simulink model "Neurofeedback_PID_WithoutFNIRS.slx"  (R2021b)
settings: Solver=ode23tb  StartTime=0.0  StopTime=30  FixedStep=0.09  RelTol=1e-8
libraries: slpidlib x1
settings Model: Creator=mdls3  LastModifiedBy=mariodelossantos
settings SolverCC: ZeroCrossControl=EnableAll
settings DebuggingCC: UnderSpecifiedDimensionMsg=warning

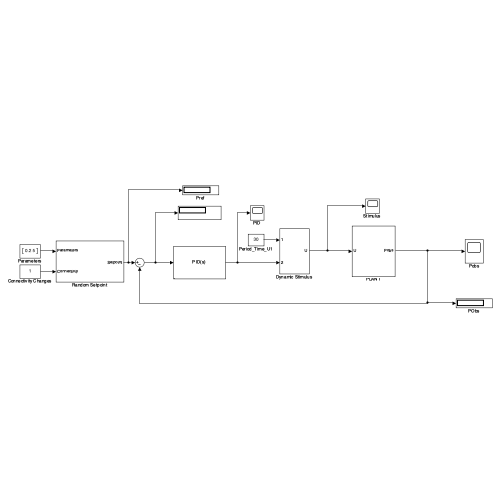
[thumbnail: Simulink's stored preview of the top-level diagram]
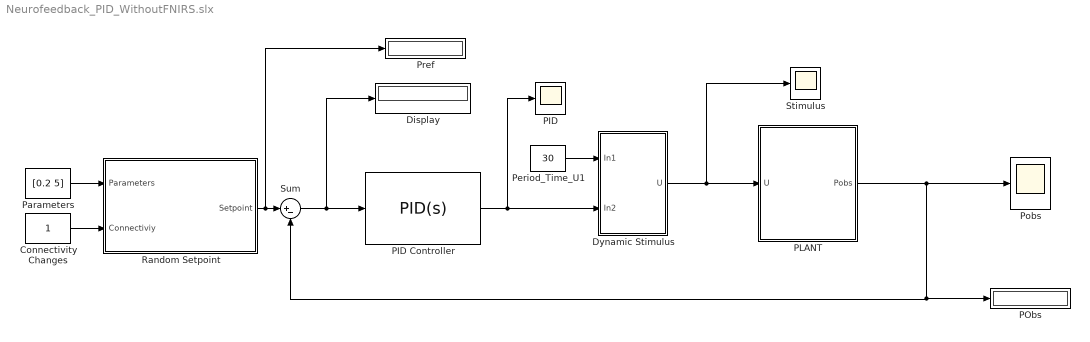
== system Neurofeedback_PID_WithoutFNIRS.slx ==
  Connectivity Changes : Constant
  Display : Display
  Dynamic Stimulus : Subsystem
  PID : Scope
  PID Controller : slpidlib/PID Controller  Controller=PID  Form=Ideal  TimeDomain=Continuous-time  UseExternalTs=off  SampleTime=-1  IntegratorMethod=Forward Euler  FilterMethod=Forward Euler  ControllerParametersSource=internal  P=0.87  I=0.1525  D=0.105  UseFilter=on  N=100  TunerSelectOption=Transfer Function Based (PID Tuner App)  InitialConditionSource=internal  InitialConditionForIntegrator=1  InitialConditionForFilter=0  DifferentiatorICPrevScaledInput=0  ExternalReset=none  TrackingMode=off  Kt=1  LimitOutput=off  SatLimitsSource=internal  UpperSaturationLimit=inf  LowerSaturationLimit=-inf  LinearizeAsGain=on  AntiWindupMode=none  Kb=1  POutMin=[]  POutMax=[]  IOutMin=[]  IOutMax=[]  DOutMin=[]  DOutMax=[]  NOutMin=[]  NOutMax=[]  SumOutMin=[]  SumOutMax=[]  SaturationOutMin=[]  SaturationOutMax=[]  PParamMin=[]  PParamMax=[]  IParamMin=[]  IParamMax=[]  DParamMin=[]  DParamMax=[]  NParamMin=[]  NParamMax=[]  KbParamMin=[]  KbParamMax=[]  KtParamMin=[]  KtParamMax=[]  KbOutMin=[]  KbOutMax=[]  KtOutMin=[]  KtOutMax=[]  IntegratorOutMin=[]  IntegratorOutMax=[]  FilterOutMin=[]  FilterOutMax=[]  SumI1OutMin=[]  SumI1OutMax=[]  SumI2OutMin=[]  SumI2OutMax=[]  SumI3OutMin=[]  SumI3OutMax=[]  SumI4OutMin=[]  SumI4OutMax=[]  SumDOutMin=[]  SumDOutMax=[]  DifferentiatorOutMin=[]  DifferentiatorOutMax=[]  FilterDiffOutCoefMin=[]  FilterDiffOutCoefMax=[]  ReciprocalOutMin=[]  ReciprocalOutMax=[]  SumDenOutMin=[]  SumDenOutMax=[]  SumNumOutMin=[]  SumNumOutMax=[]  DivideOutMin=[]  DivideOutMax=[]  UdiffTsProdOutMin=[]  UdiffTsProdOutMax=[]  NTsProdOutMin=[]  NTsProdOutMax=[]  UintegralTsProdOutMin=[]  UintegralTsProdOutMax=[]  UngainTsProdOutMin=[]  UngainTsProdOutMax=[]  IntegratorContinuousStateAttributes=''  IntegratorStateMustResolveToSignalObject=off  IntegratorRTWStateStorageClass=Auto  FilterContinuousStateAttributes=''  FilterStateMustResolveToSignalObject=off  FilterRTWStateStorageClass=Auto  ParallelPVariant=Passthrough  IdealPVariant=InternalParameters  IVariant=InternalParameters  DVariant=InternalParameters  IntegratorVariant=Continuous  SatVariant=Disabled  AWVariant=Passthrough  PCopyVariant=Disabled  TRVariant=Disabled  FdbkBlocksVariant=Forward  IdealPFdbkVariant=Disabled  SatFdbkVariant=Disabled  DerivativeFilterVariant=ContFilter  NVariant=InternalParameters  NCopyVariant=Disabled  FilterICVariant=InternalICsFilter  IntegratorICVariant=InternalICs  ExternalResetVariant=Disabled  TRSumVariant=Passthrough  SumFdbkVariant=Disabled  SumVariant=Sum_PID  TsampFilterVariant=InternalTs  TsampNgainVariant=Passthrough  TsampIntegralVariant=Passthrough  ExternalSaturationOutDataTypeStr=Inherit: Same as second input
  PLANT : Subsystem
  PObs : Display
  Parameters : Constant  Value=[0.2 5]
  Period_Time_U1 : Constant  Value=30
  Pobs : Scope
  Pref : Display
  Random Setpoint : Subsystem
  Stimulus : Scope
  Sum : Sum  Inputs=|+-
  wires:
  Period_Time_U1/1 -> Dynamic Stimulus/1(In1)
  Dynamic Stimulus/1(U) -> Stimulus/1, PLANT/1(U)
  PID Controller/1 -> Dynamic Stimulus/2(In2), PID/1
  Sum/1 -> PID Controller/1, Display/1
  PLANT/1(Pobs) -> Pobs/1, Sum/2, PObs/1
  Parameters/1 -> Random Setpoint/1(Parameters)
  Random Setpoint/1(Setpoint) -> Pref/1, Sum/1
  Connectivity Changes/1 -> Random Setpoint/2(Connectiviy)

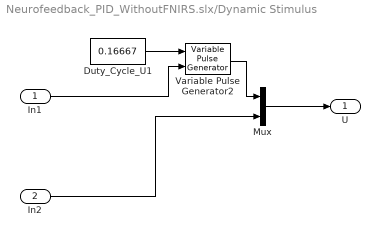
== system Neurofeedback_PID_WithoutFNIRS.slx/Dynamic Stimulus ==
  In1 : Inport
  In2 : Inport  Port=2
  Duty_Cycle_U1 : Constant  Value=0.16667  OutMin=[0]  OutMax=[0.8]
  Mux : Mux  Inputs=2
  Variable Pulse Generator2 : VariablePulseGenerator  RunAtFixedTimeIntervals=on  SampleTime=1/10.4
  U : Outport
  wires:
  In1/1 -> Variable Pulse Generator2/2
  Mux/1 -> U/1
  Variable Pulse Generator2/1 -> Mux/1
  Duty_Cycle_U1/1 -> Variable Pulse Generator2/1
  In2/1 -> Mux/2

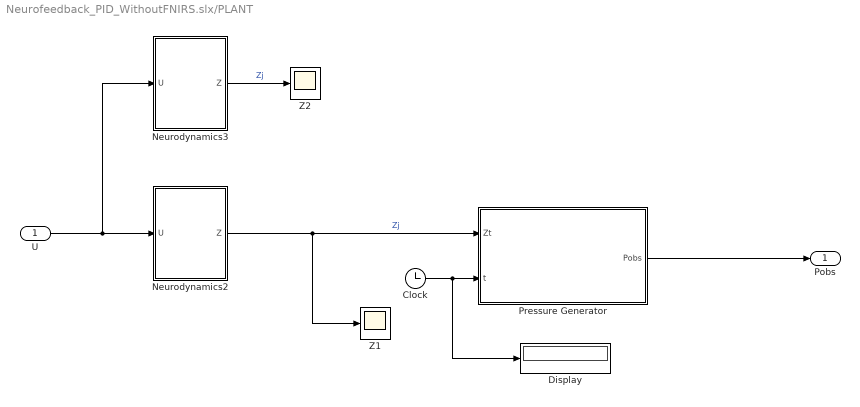
== system Neurofeedback_PID_WithoutFNIRS.slx/PLANT ==
  U : Inport
  Clock : Clock
  Display : Display
  Neurodynamics2 : Subsystem
  Neurodynamics3 : Subsystem
  Pressure Generator : MATLAB Function  TreatAsAtomicUnit=on
  Z1 : Scope
  Z2 : Scope
  Pobs : Outport
  wires:
  Clock/1 -> Display/1, Pressure Generator/2(t)
  Pressure Generator/1(Pobs) -> Pobs/1
  Neurodynamics2/1(Z) -> Z1/1, Pressure Generator/1(Zt)  "Zj"
  U/1 -> Neurodynamics3/1(U), Neurodynamics2/1(U)
  Neurodynamics3/1(Z) -> Z2/1  "Zj"

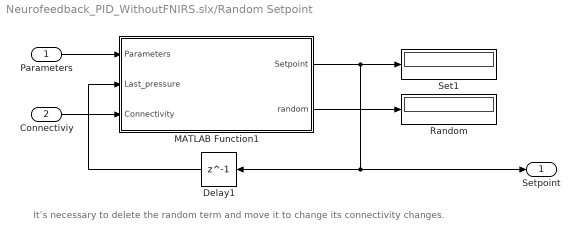
== system Neurofeedback_PID_WithoutFNIRS.slx/Random Setpoint ==
  note: It’s necessary to delete the random term and move it to change its connectivity changes.
  Parameters : Inport
  Connectiviy : Inport  Port=2
  Delay1 : Delay  DelayLength=1  InitialCondition=0
  MATLAB Function1 : MATLAB Function  TreatAsAtomicUnit=on
  Random : Display
  Set1 : Display
  Setpoint : Outport
  wires:
  Parameters/1 -> MATLAB Function1/1(Parameters)
  MATLAB Function1/2(random) -> Random/1
  MATLAB Function1/1(Setpoint) -> Set1/1, Setpoint/1, Delay1/1
  Delay1/1 -> MATLAB Function1/2(Last_pressure)
  Connectiviy/1 -> MATLAB Function1/3(Connectivity)

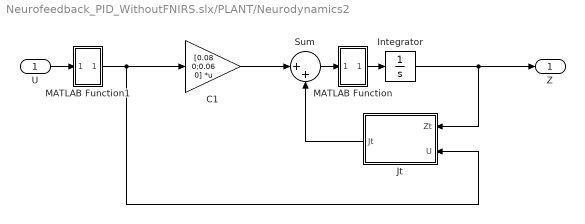
== system Neurofeedback_PID_WithoutFNIRS.slx/PLANT/Neurodynamics2 ==
  U : Inport
  C1 : Gain  Gain=[0.08 0;0.06 0]  Multiplication=Matrix(K*u) (u vector)
  Integrator : Integrator
  Jt : MATLAB Function  TreatAsAtomicUnit=on
  MATLAB Function : MATLAB Function  TreatAsAtomicUnit=on
  MATLAB Function1 : MATLAB Function  TreatAsAtomicUnit=on
  Sum : Sum  Inputs=|++
  Z : Outport
  wires:
  Integrator/1 -> Z/1, Jt/1(Zt)
  C1/1 -> Sum/1
  Jt/1(Jt) -> Sum/2
  U/1 -> MATLAB Function1/1(Z)
  Sum/1 -> MATLAB Function/1(Z)
  MATLAB Function1/1(Zn) -> C1/1, Jt/2(U)
  MATLAB Function/1(Zn) -> Integrator/1

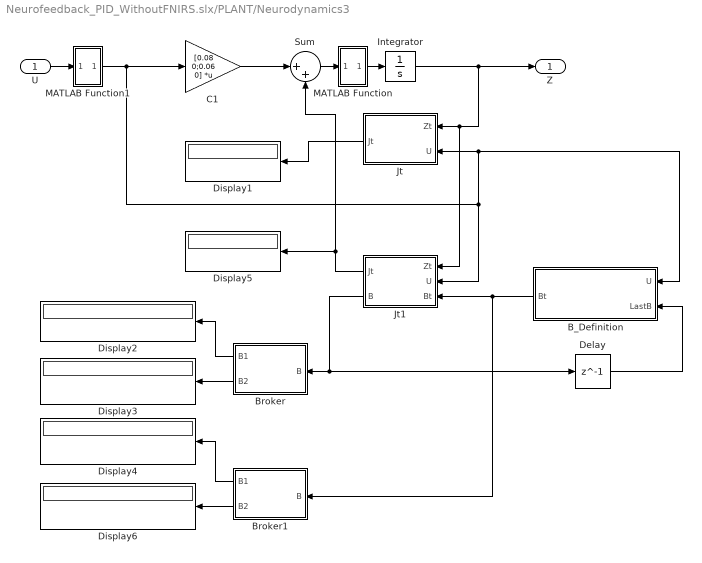
== system Neurofeedback_PID_WithoutFNIRS.slx/PLANT/Neurodynamics3 ==
  U : Inport
  B_Definition : MATLAB Function  TreatAsAtomicUnit=on
  Broker : MATLAB Function  TreatAsAtomicUnit=on
  Broker1 : MATLAB Function  TreatAsAtomicUnit=on
  C1 : Gain  Gain=[0.08 0;0.06 0]  Multiplication=Matrix(K*u) (u vector)
  Delay : Delay  DelayLength=1  InitialCondition=0
  Display{1..6} (6 alike) : Display
  Integrator : Integrator
  Jt : MATLAB Function  TreatAsAtomicUnit=on
  Jt1 : MATLAB Function  TreatAsAtomicUnit=on
  MATLAB Function : MATLAB Function  TreatAsAtomicUnit=on
  MATLAB Function1 : MATLAB Function  TreatAsAtomicUnit=on
  Sum : Sum  Inputs=|++
  Z : Outport
  wires:
  Integrator/1 -> Z/1, Jt1/1(Zt), Jt/1(Zt)
  C1/1 -> Sum/1
  Jt/1(Jt) -> Display1/1
  U/1 -> MATLAB Function1/1(Z)
  Sum/1 -> MATLAB Function/1(Z)
  MATLAB Function1/1(Zn) -> C1/1, Jt1/2(U), B_Definition/1(U), Jt/2(U)
  MATLAB Function/1(Zn) -> Integrator/1
  Jt1/1(Jt) -> Sum/2, Display5/1
  Delay/1 -> B_Definition/2(LastB)
  Jt1/2(B) -> Broker/1(B), Delay/1
  Broker/1(B1) -> Display2/1
  Broker/2(B2) -> Display3/1
  B_Definition/1(Bt) -> Broker1/1(B), Jt1/3(Bt)
  Broker1/2(B2) -> Display6/1
  Broker1/1(B1) -> Display4/1

== matlab function Neurofeedback_PID_WithoutFNIRS.slx/PLANT/Neurodynamics3/MATLAB Function1 ==
  data: Z input; Zn output
function Zn = fcn(Z)

Zn = Z(:,1);

== matlab function Neurofeedback_PID_WithoutFNIRS.slx/PLANT/Pressure Generator ==
  data: Zt input; Pobs output; t input
function Pobs = fcn(Zt, t)
    R=28.2; %Resistor [Ohms];
    C=0.8; %Capacitor [Faradays];
    V= Zt(1,:); %Voltage or system reference;
    Vc = V * (exp(-t/(R*C))); % Voltage at the capacitor  
    
Pobs = Vc;

== matlab function Neurofeedback_PID_WithoutFNIRS.slx/Random Setpoint/MATLAB Function1 ==
  settings: updateMethod=DISCRETE
  data: Setpoint output; Parameters input; Last_pressure input; random output; Connectivity input
function [Setpoint, random] = Random_Setpoint(Parameters, Last_pressure, Connectivity)
    %Parameters = [threshold Start_setpoint]
    temp = 0;
   %Pressure Setpoint selection
    pmin = 4;
    pmax = 8;
    new_pressure = pmin + rand(1)*(pmax-pmin);

    %Random used to simulate the connectivity changes, so we must change
    %the pressure setpoint when changes in the connectitvy are observed.
    min = 0;
    tmax = 10;
        %We should fine a random criteria to change the setpoint, not just
        %time, or the moment B changes. For now works to demostrate the
        %control without fNIRS
    random = min + rand(1) * (tmax - min) * new_pressure;
    if (Connectivity == 1)
         if (random < Parameters(1))
            %disp("Time")
            %disp(Time)
            temp = new_pressure;
            %disp("Setpoint")
            %disp(temp)
        else 
            temp = Last_pressure;
                if (Parameters(2) == temp || temp == 0)
                    temp = Parameters(2);
                else
                    temp = Last_pressure;
                end
         end  
    else
        temp = Parameters(2);
    end

    Setpoint = temp;

== matlab function Neurofeedback_PID_WithoutFNIRS.slx/PLANT/Neurodynamics3/Broker ==
  data: B input; B1 output; B2 output
function [B1, B2] = fcn(B)
B1 = B(:,:,1);
B2 = B(:,:,2);

== matlab function Neurofeedback_PID_WithoutFNIRS.slx/PLANT/Neurodynamics2/MATLAB Function1 ==
  data: Z input; Zn output
function Zn = fcn(Z)

Zn = Z(:,1);

== matlab function Neurofeedback_PID_WithoutFNIRS.slx/PLANT/Neurodynamics2/MATLAB Function ==
  data: Z input; Zn output
function Zn = fcn(Z)

Zn = Z(:,1);

== matlab function Neurofeedback_PID_WithoutFNIRS.slx/PLANT/Neurodynamics3/Broker1 ==
  data: B input; B1 output; B2 output
function [B1, B2] = fcn(B)
B1 = B(:,:,1);
B2 = B(:,:,2);

== matlab function Neurofeedback_PID_WithoutFNIRS.slx/PLANT/Neurodynamics3/Jt1 ==
  data: Zt input; U input; Jt output; Bt input; B output
function [Jt, B] = fcn(Zt, U, Bt)

   A = [-0.16 -0.49;-0.02 -0.33];
   nRegions  = size(A,1);

   B = zeros(2,2,2);
   a = 0;
   B1 = [0 0; 0 0]; %There must be a B per stimulus
   B2 = [-0.02 -0.77; 0.33 -1.31];

   if Bt(:,:,2) ~= B(:,:,2)
       B(:,:,:) = Bt(:,:,:);
   else
          B(:,:,1) = B1;
          B(:,:,2) = B2;
   end
   M = size(U,1); %nStimuli
   assert(M == size(B,3),...
        'Unexpected number of induced connectivity parameters B.');



   T = zeros(nRegions); %nRegions x nRegions
               for uu = 1:M % Sum (Uj * Bj)
                   tmp = U(uu,:) * B(:,:,uu);
                   T = -0.5 * exp(T + tmp);  
               end
        SI = diag(A);
        A =  A - diag(exp(SI) + (SI));
Jt = (A*Zt) + (T*Zt);

== matlab function Neurofeedback_PID_WithoutFNIRS.slx/PLANT/Neurodynamics3/B_Definition ==
  settings: updateMethod=DISCRETE
  data: U input; Bt output; LastB input
function Bt = B_Definition(U, LastB)
    Bt = zeros(2, 2, 2);
   %Control extraction and weight
   Ucontrol = U(2) * (0 + rand(1) * 1);
   Threshold = 0.2;
    if(Ucontrol < Threshold) %Random Ucontrol to test
        min = -2; 
        max = 2;
        n = 2;
        r1 = min + rand(n)*(max-min);
        r2 = min + rand(n)*(max-min);
        %Bt(:,:,1) = r1(:,:);
        Bt(:,:,2) = r2(:,:);
    else
       Bt = LastB;
    end

== matlab function Neurofeedback_PID_WithoutFNIRS.slx/PLANT/Neurodynamics3/Jt ==
  data: Zt input; U input; Jt output
function Jt = fcn(Zt, U)
   A = [-0.16 -0.49;-0.02 -0.33];
   nRegions  = size(A,1);
   M = size(U,1); %nStimuli
   simulationLength = size(U,2);
   B = zeros(2,2,2);
   B1 = [0 0; 0 0]; %There must be a B per stimulus
   B2 = [-0.02 -0.77; 0.33 -1.31];
   B(:,:,1) = B1;
   B(:,:,2) = B2;
      assert(M == size(B,3),...
       'Unexpected number of induced connectivity parameters B.');
   T = zeros(nRegions); %nRegions x nRegions
    for t = 1:simulationLength
           for uu = 1:M % Sum (Uj * Bj)
               tmp = U(uu,t)*B(:,:,uu);
               T = -0.5*exp(T + tmp);  
           end
    end
    SI = diag(A);
    A =  A - diag(exp(SI) + (SI));
Jt = (A*Zt) + (T*Zt);

== matlab function Neurofeedback_PID_WithoutFNIRS.slx/PLANT/Neurodynamics2/Jt ==
  data: Zt input; U input; Jt output
function Jt = fcn(Zt, U)
   A = [-0.16 -0.49;-0.02 -0.33];
   nRegions  = size(A,1);
   M = size(U,1); %nStimuli
   simulationLength = size(U,2);
   B = zeros(2,2,2);
   B1 = [0 0; 0 0]; %There must be a B per stimulus
   B2 = [-0.02 -0.77; 0.33 -1.31];
   B(:,:,1) = B1;
   B(:,:,2) = B2;
      assert(M == size(B,3),...
       'Unexpected number of induced connectivity parameters B.');
   T = zeros(nRegions); %nRegions x nRegions
    for t = 1:simulationLength
           for uu = 1:M % Sum (Uj * Bj)
               tmp = U(uu,t)*B(:,:,uu);
               T = -0.5*exp(T + tmp);  
           end
    end
    SI = diag(A);
    A =  A - diag(exp(SI) + (SI));
Jt = (A*Zt) + (T*Zt);

== matlab function Neurofeedback_PID_WithoutFNIRS.slx/PLANT/Neurodynamics3/MATLAB Function ==
  data: Z input; Zn output
function Zn = fcn(Z)

Zn = Z(:,1);
